simulink subsystem "a2v"  (R2021b)
settings: Solver=VariableStepAuto  StartTime=0.0  StopTime=10.0  RelTol=1e-3
settings Model: Creator=yurid  LastModifiedBy=yurid

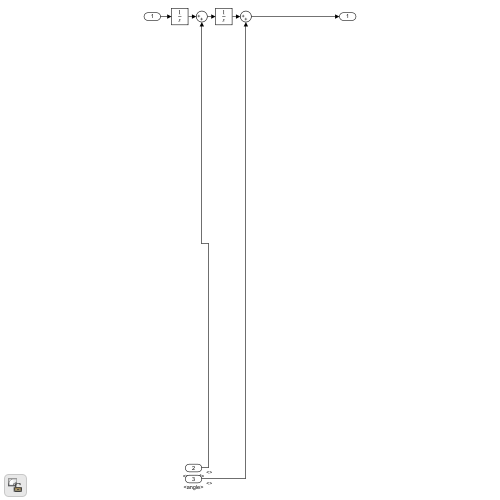
[thumbnail: Simulink's stored preview of the top-level diagram]
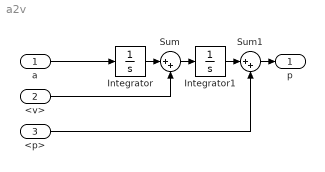
== system a2v ==
  a : Inport
  <v> : Inport  Port=2
  <p> : Inport  Port=3
  Integrator : Integrator
  Integrator1 : Integrator
  Sum : Sum  Inputs=|++
  Sum1 : Sum  Inputs=|++
  p : Outport
  wires:
  Integrator1/1 -> Sum1/1
  a/1 -> Integrator/1
  <v>/1 -> Sum/2
  Integrator/1 -> Sum/1
  Sum/1 -> Integrator1/1
  <p>/1 -> Sum1/2
  Sum1/1 -> p/1
